simulink model "Simhinf"  (R2016b)
settings: Solver=FixedStepAuto  StartTime=0.0  StopTime=simTime  FixedStep=Ts  RelTol=1e-3
values from neighbouring files (symbols this model uses):
  xinit = (pi/180)*[3 3 0 0 3 3 0 0]    [EEN050_lab_preparation.m]
undefined symbols (not defined in the file or in its folder): ah, bh, ch, dh, Pnom
libraries: simulink_extras x1
settings Model: ExtModeTrigDuration=120000  Creator=MLevis  LastModifiedBy=labb2
settings SolverCC: PositivePriorityOrder=on
settings DataIOCC: SaveFormat=StructureWithTime  SignalLoggingSaveFormat=ModelDataLogs
settings OptimizationCC: BooleanDataType=off  OptimizeBlockIOStorage=off  BufferReuse=off  GlobalBufferReuse=off  ExpressionFolding=off  ExpressionDepthLimit=2147483647  LocalBlockOutputs=off  InitFltsAndDblsToZero=on  LifeSpan=inf
settings DebuggingCC: SaveWithParameterizedLinksMsg=none  UnderspecifiedInitializationDetection=Classic  MergeDetectMultiDrivingBlocksExec=none  SignalResolutionControl=TryResolveAllWithWarning  MultiTaskDSMMsg=warning  FcnCallInpInsideContextMsg=warning  StateNameClashWarn=warning  SFUnexpectedBacktrackingDiag=warning  SFNoUnconditionalDefaultTransitionDiag=warning  SFExecutionAtInitializationDiag=none
settings HardwareCC: ProdBitPerPointer=32  ProdBitPerSizeT=32  ProdBitPerPtrDiffT=32  ProdLargestAtomicFloat=None  ProdIntDivRoundTo=Undefined  ProdEndianess=Unspecified  ProdWordSize=32  ProdHWDeviceType=32-bit Generic  TargetHWDeviceType=32-bit Generic
settings ModelReferenceCC: PropagateSignalLabelsOutOfModel=off
settings RTWCC: SystemTargetFile=quarc_win64.tlc  TemplateMakefile=quarc_default_tmf  Description=QUARC Win64 Target
settings STFCustomTargetCC: TargetPreCompLibLocation=C:\PROGRA~3\QUARC\lib\2016b\win64\release  ConcurrentExecutionCompliant=on  GeneratePreprocessorConditionals=Disable all  CPPClassGenCompliant=on  SystemTargetFile=quarc_win64.tlc
settings GRTTargetCC: TargetPreCompLibLocation=C:\PROGRA~3\QUARC\lib\2016b\win64\release  TargetLangStandard=C89/C90 (ANSI)  ParMdlRefBuildCompliant=off  CompOptLevelCompliant=off  GeneratePreprocessorConditionals=Disable all  CombineOutputUpdateFcns=off  MatFileLogging=off  GRTInterface=on  UseToolchainInfoCompliant=off  ExtMode=on  ExtModeMexFile=quarc_comm
settings ConfigComp: CovMetricSettings=dw  CovHtmlReporting=on  CovSaveCumulativeToWorkspaceVar=on  CovSaveSingleToWorkspaceVar=on  CovExternalEMLEnable=off

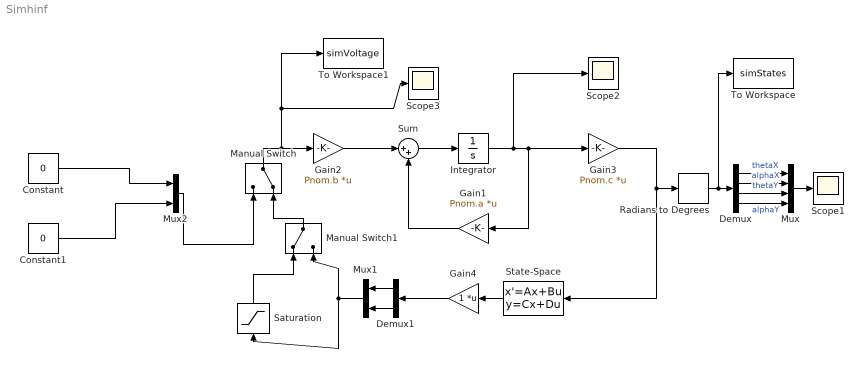
== system Simhinf ==
  Constant : Constant  Value=0
  Constant1 : Constant  Value=0
  Demux : Demux
  Demux1 : Demux  Outputs=2
  Gain1 : Gain  Gain=Pnom.a  Multiplication=Matrix(K*u) (u vector)
  Gain2 : Gain  Gain=Pnom.b  Multiplication=Matrix(K*u) (u vector)
  Gain3 : Gain  Gain=Pnom.c  Multiplication=Matrix(K*u) (u vector)
  Gain4 : Gain  Multiplication=Matrix(K*u)
  Integrator : Integrator  InitialCondition=xinit
  Manual Switch : ManualSwitch  CurrentSetting=0
  Manual Switch1 : ManualSwitch
  Mux : Mux
  Mux1 : Mux  Inputs=2
  Mux2 : Mux  Inputs=2
  Radians to Degrees : simulink_extras/Transformations/Radians to Degrees
  Saturation : Saturate  UpperLimit=10  LowerLimit=-10
  Scope1 : Scope
  Scope2 : Scope
  Scope3 : Scope
  State-Space : StateSpace  A=ah  B=bh  C=ch  D=dh  X0=0
  Sum : Sum  Inputs=|++
  To Workspace : ToWorkspace  VariableName=simStates  SaveFormat=Timeseries  SampleTime=-1
  To Workspace1 : ToWorkspace  VariableName=simVoltage  SaveFormat=Timeseries  SampleTime=-1
  wires:
  Integrator/1 -> Scope2/1, Gain1/1, Gain3/1
  Gain1/1 -> Sum/2
  Gain2/1 -> Sum/1
  Sum/1 -> Integrator/1
  Demux/1 -> Mux/1  "thetaX"
  Demux/2 -> Mux/2  "alphaX"
  Demux/3 -> Mux/3  "thetaY"
  Demux/4 -> Mux/4  "alphaY"
  Mux/1 -> Scope1/1
  Radians to Degrees/1 -> To Workspace/1, Demux/1
  State-Space/1 -> Gain4/1
  Mux1/1 -> Manual Switch1/2, Saturation/1
  Demux1/1 -> Mux1/1
  Demux1/2 -> Mux1/2
  Saturation/1 -> Manual Switch1/1
  Manual Switch/1 -> Scope3/1, To Workspace1/1, Gain2/1
  Mux2/1 -> Manual Switch/1
  Constant/1 -> Mux2/1
  Constant1/1 -> Mux2/2
  Manual Switch1/1 -> Manual Switch/2
  Gain3/1 -> State-Space/1, Radians to Degrees/1
  Gain4/1 -> Demux1/1
